simulink model "Alex_SERGIO_wrist"  (R2016b)
settings: Solver=FixedStepDiscrete  StartTime=0.0  StopTime=3600  FixedStep=1/1000  RelTol=1e-3  EnableMultiTasking=on
values from neighbouring files (symbols this model uses):
  abs2deg_s1 = (s1max-s1min)/(s1maxabs-s1minabs)    (= 0.280034572169)    [Alex_init_const_wrist.m]
  abs2deg_s2 = (s2max-s2min)/(s2maxabs-s2minabs)    (= 0.060826446281)    [Alex_init_const_wrist.m]
  ilim_w1 = 1.0    (= 1)    [Alex_init_const_wrist.m]
  ilim_w2 = 1.0    (= 1)    [Alex_init_const_wrist.m]
  Kd_w1 = 0.0    (= 0)    [Alex_init_const_wrist.m]
  Kd_w2 = 0.0    (= 0)    [Alex_init_const_wrist.m]
  Ki_w1 = 0.0    (= 0)    [Alex_init_const_wrist.m]
  Ki_w2 = 0.0    (= 0)    [Alex_init_const_wrist.m]
  s1maxabs = 2374    [Alex_init_const_wrist.m]
  s1minabs = 1217    [Alex_init_const_wrist.m]
  s2maxabs = 3420    [Alex_init_const_wrist.m]
  s2minabs = 395    [Alex_init_const_wrist.m]
  Ts = 1/Fs    [Alex_init_const_shoulderelbow.m]    (also in Alex_init_const_wrist.m = 0.001)
undefined symbols (not defined in the file or in its folder): CPT_w1, CPT_w2, GR_w1, GR_w2
libraries: SERGIOarm x4, SERGIO_Lib x1
settings Model: SimulationMode=external  ExtModeTrigElement=1  ExtModeTrigDuration=3910  ExtModeAutoUpdateStatusClock=off  Creator=root  LastModifiedBy=Matthijs
settings DataIOCC: MaxDataPoints=4000*3600  SaveFormat=Array  SignalLoggingSaveFormat=ModelDataLogs  SaveOutput=off  SignalLogging=off  SaveTime=off
settings OptimizationCC: BlockReduction=off  BooleanDataType=off  ExpressionDepthLimit=2147483647  InitFltsAndDblsToZero=on  LifeSpan=inf
settings DebuggingCC: SaveWithParameterizedLinksMsg=none  UnderspecifiedInitializationDetection=Classic  MergeDetectMultiDrivingBlocksExec=none  SignalResolutionControl=TryResolveAllWithWarning  MultiTaskDSMMsg=warning  MultiTaskCondExecSysMsg=none  FcnCallInpInsideContextMsg=warning  StateNameClashWarn=warning  StrictBusMsg=None  SFUnexpectedBacktrackingDiag=warning  SFNoUnconditionalDefaultTransitionDiag=warning  SFExecutionAtInitializationDiag=none
settings HardwareCC: ProdBitPerPointer=32  ProdBitPerSizeT=32  ProdBitPerPtrDiffT=32  ProdLargestAtomicFloat=None  ProdIntDivRoundTo=Undefined  ProdEndianess=Unspecified  ProdWordSize=32  ProdHWDeviceType=32-bit Generic  TargetBitPerPointer=64  TargetBitPerSizeT=64  TargetBitPerPtrDiffT=64  TargetLongLongMode=on  TargetIntDivRoundTo=Zero  TargetEndianess=LittleEndian  TargetWordSize=64  TargetHWDeviceType=MATLAB Host
settings ModelReferenceCC: ModelReferencePassRootInputsByReference=off  PropagateSignalLabelsOutOfModel=off
settings RTWCC: SystemTargetFile=mttarget.tlc  MakeCommand="make_rtw CC=\"ccache gcc\" OPTS=\"-DNETIF_ID=0 -D_GNU_SOURCE -DPRIO=99\""  TemplateMakefile=mt_unix.tmf  Description=Robocup Real-Time Motion Target  RTWCompilerOptimization=Custom  RTWCustomCompilerOptimizations=-O2 -g -W
settings RTWCC: CustomInclude=|
  | /usr/local/include/soem
  | /usr/local/include/timer_posix
settings RTWCC: CustomLibrary=|
  | /usr/local/lib/libsoem.so
  | /usr/lib/libtimer_posix.so
settings GRTTargetCC: TargetLangStandard=C89/C90 (ANSI)  GeneratePreprocessorConditionals=Disable all  UseToolchainInfoCompliant=off  ExtMode=on
settings ConfigComp: CovMetricSettings=dw  CovHtmlReporting=on  CovSaveCumulativeToWorkspaceVar=on  CovSaveSingleToWorkspaceVar=on  CovExternalEMLEnable=off

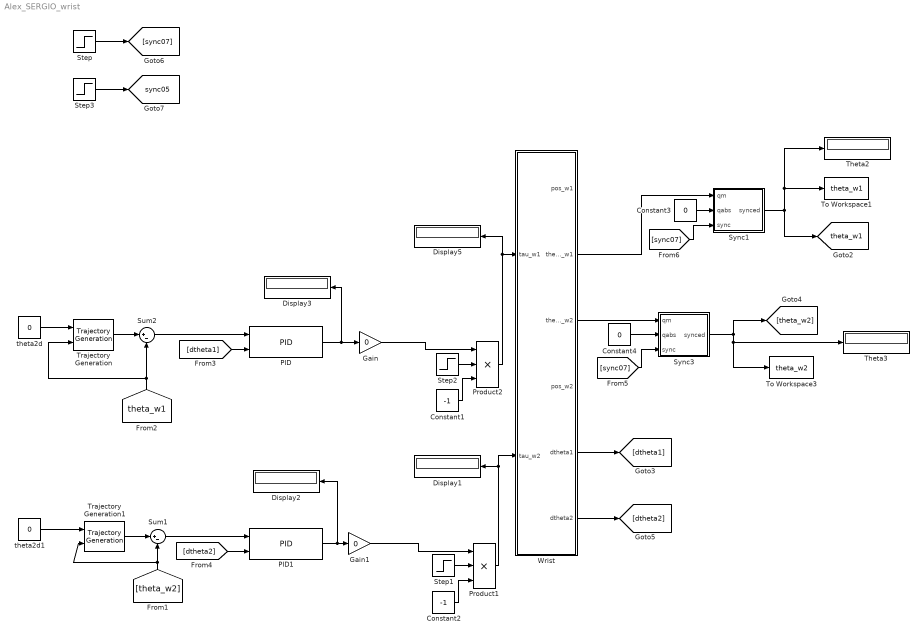
== system Alex_SERGIO_wrist ==
  Constant1 : Constant  Value=-1
  Constant2 : Constant  Value=-1
  Constant3 : Constant  Value=0
  Constant4 : Constant  Value=0
  Display{1..3,5} (4 alike) : Display
  Gain : Gain  Gain=0
  Gain1 : Gain  Gain=0
  PID : SERGIOarm/PID  Kc=Kc_w1  Ki=Ki_w1  Kd=Kd_w1  uplim=ilim_w1  lowlim=-ilim_w1  Ts=Ts
  PID1 : SERGIOarm/PID  Kc=Kc_w2  Ki=Ki_w2  Kd=Kd_w2  uplim=ilim_w2  lowlim=-ilim_w2  Ts=Ts
  Product1 : Product  Inputs=3  RndMeth=Zero
  Product2 : Product  Inputs=3  RndMeth=Zero
  Step : Step  Time=0.7  Before=1  After=0  SampleTime=0
  Step1 : Step  Time=0.8  After=0  SampleTime=0
  Step2 : Step  Time=0.8  After=0  SampleTime=0
  Step3 : Step  Time=0.5  Before=1  After=0  SampleTime=0
  Sum1 : Sum  Inputs=|+-
  Sum2 : Sum  Inputs=|+-
  Sync1 : Subsystem
  Sync3 : Subsystem
  Theta2 : Display
  Theta3 : Display
  To Workspace1 : ToWorkspace  VariableName=theta_w1  SampleTime=-1
  To Workspace3 : ToWorkspace  VariableName=theta_w2  SampleTime=-1
  Trajectory Generation : SERGIOarm/Trajectory Generation  Vmax=0  Amax=0  dif_in=0
  Trajectory Generation1 : SERGIOarm/Trajectory Generation  Vmax=0  Amax=0  dif_in=0
  Wrist : Subsystem
  theta2d : Constant  Value=0
  theta2d1 : Constant  Value=0
  tag scope: sync05=global, theta_w1=global
  wires:
  [theta_w1] -> Sum2/2, Trajectory Generation/2
  Product2/1 -> Wrist/1(tau_w1), Display5/1
  Step/1 -> [sync07]
  Step3/1 -> [sync05]
  Step2/1 -> Product2/2
  Constant1/1 -> Product2/3
  [dtheta1] -> PID/2
  [theta_w2] -> Sum1/2, Trajectory Generation1/2
  Product1/1 -> Display1/1, Wrist/2(tau_w2)
  Step1/1 -> Product1/2
  Constant2/1 -> Product1/3
  [dtheta2] -> PID1/2
  Sync3/1(synced) -> [theta_w2], Theta3/1, To Workspace3/1
  [sync07] -> Sync3/3(sync)
  Sum1/1 -> PID1/1
  [sync07] -> Sync1/3(sync)
  Sync1/1(synced) -> [theta_w1], To Workspace1/1, Theta2/1
  Wrist/2(theta_w1) -> Sync1/1(qm)
  Constant3/1 -> Sync1/2(qabs)
  Wrist/3(theta_w2) -> Sync3/1(qm)
  Constant4/1 -> Sync3/2(qabs)
  Wrist/6(dtheta2) -> [dtheta2]
  Wrist/5(dtheta1) -> [dtheta1]
  PID/1 -> Gain/1, Display3/1
  Gain/1 -> Product2/1
  PID1/1 -> Gain1/1, Display2/1
  Gain1/1 -> Product1/1
  theta2d/1 -> Trajectory Generation/1
  Trajectory Generation/1 -> Sum2/1
  Sum2/1 -> PID/1
  Trajectory Generation1/1 -> Sum1/1
  theta2d1/1 -> Trajectory Generation1/1

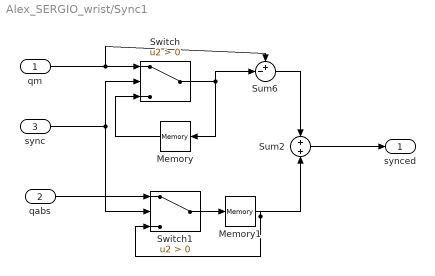
== system Alex_SERGIO_wrist/Sync1 ==
  qm : Inport
  qabs : Inport  Port=2
  sync : Inport  Port=3
  Memory : Memory
  Memory1 : Memory
  Sum2 : Sum
  Sum6 : Sum  Inputs=+-|
  Switch : Switch  Criteria=u2 > Threshold
  Switch1 : Switch  Criteria=u2 > Threshold
  synced : Outport
  wires:
  Switch/1 -> Sum6/2, Memory/1
  Memory/1 -> Switch/3
  qm/1 -> Switch/1, Sum6/1
  Sum6/1 -> Sum2/1
  Sum2/1 -> synced/1
  sync/1 -> Switch/2, Switch1/2
  Memory1/1 -> Switch1/3, Sum2/2
  Switch1/1 -> Memory1/1
  qabs/1 -> Switch1/1

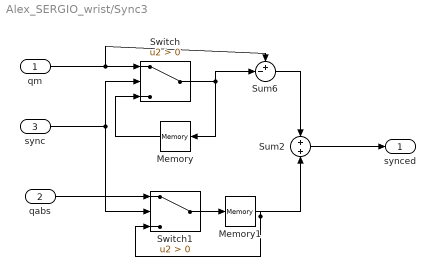
== system Alex_SERGIO_wrist/Sync3 ==
  qm : Inport
  qabs : Inport  Port=2
  sync : Inport  Port=3
  Memory : Memory
  Memory1 : Memory
  Sum2 : Sum
  Sum6 : Sum  Inputs=+-|
  Switch : Switch  Criteria=u2 > Threshold
  Switch1 : Switch  Criteria=u2 > Threshold
  synced : Outport
  wires:
  Switch/1 -> Sum6/2, Memory/1
  Memory/1 -> Switch/3
  qm/1 -> Switch/1, Sum6/1
  Sum6/1 -> Sum2/1
  Sum2/1 -> synced/1
  sync/1 -> Switch/2, Switch1/2
  Memory1/1 -> Switch1/3, Sum2/2
  Switch1/1 -> Memory1/1
  qabs/1 -> Switch1/1

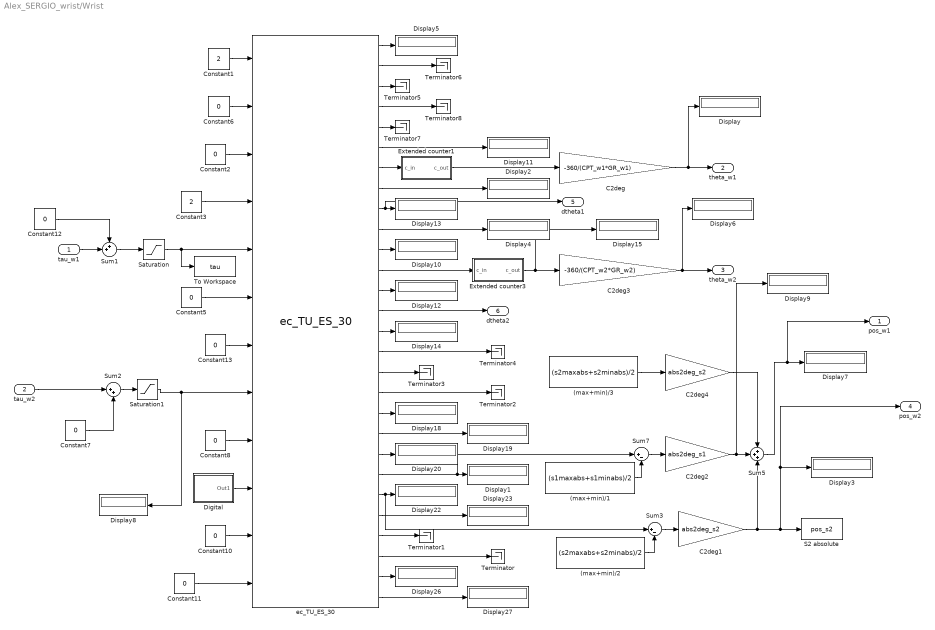
== system Alex_SERGIO_wrist/Wrist ==
  tau_w1 : Inport
  tau_w2 : Inport  Port=2
  (max+min)/1 : Constant  Value=(s1maxabs+s1minabs)/2
  (max+min)/2 : Constant  Value=(s2maxabs+s2minabs)/2
  (max+min)/3 : Constant  Value=(s2maxabs+s2minabs)/2
  C2deg : Gain  Gain=-360/(CPT_w1*GR_w1)
  C2deg1 : Gain  Gain=abs2deg_s2
  C2deg2 : Gain  Gain=abs2deg_s1
  C2deg3 : Gain  Gain=-360/(CPT_w2*GR_w2)
  C2deg4 : Gain  Gain=abs2deg_s2
  Constant1 : Constant  Value=2
  Constant{2,5..8,10..13} (9 alike) : Constant  Value=0
  Constant3 : Constant  Value=2
  Digital : Subsystem
  Display{,1..15,18..20,22..23,26..27} (23 alike) : Display
  Extended counter1 : Subsystem
  Extended counter3 : Subsystem
  S2 absolute : ToWorkspace  VariableName=pos_s2  SampleTime=-1
  Saturation : Saturate  UpperLimit=400  LowerLimit=-400
  Saturation1 : Saturate  UpperLimit=400  LowerLimit=-400
  Sum1 : Sum  Inputs=++|
  Sum2 : Sum  Inputs=|++
  Sum3 : Sum  Inputs=|+-
  Sum5 : Sum  Inputs=+++
  Sum7 : Sum  Inputs=|+-
  Terminator{,1..8} (9 alike) : Terminator
  To Workspace : ToWorkspace  VariableName=tau  SampleTime=-1
  ec_TU_ES_30 : SERGIO_Lib/EtherCAT Blocks/ec_TU_ES_30  link_id=3  slave_num=4  resistance=[0.0, 0, 0]  kv=[0.0, 0, 0]  pgain=[0.00, 10.00, 0.00]  igain=[0.00, 5.00, 0.00]  ilimit=[1.0, 1.0, 1.0]  encdir=[1, 1, -1]  encres=[1024, 512, 512]  czero=[17230, 8835, 8775]
  pos_w1 : Outport
  theta_w1 : Outport  Port=2
  theta_w2 : Outport  Port=3
  pos_w2 : Outport  Port=4
  dtheta1 : Outport  Port=5
  dtheta2 : Outport  Port=6
  wires:
  Constant2/1 -> ec_TU_ES_30/3
  Constant5/1 -> ec_TU_ES_30/6
  Constant8/1 -> ec_TU_ES_30/9
  Digital/1(Out1) -> ec_TU_ES_30/10
  Constant10/1 -> ec_TU_ES_30/11
  Constant11/1 -> ec_TU_ES_30/12
  ec_TU_ES_30/1 -> Display5/1
  ec_TU_ES_30/3 -> Terminator5/1
  ec_TU_ES_30/5 -> Terminator7/1
  ec_TU_ES_30/6 -> Display11/1
  ec_TU_ES_30/8 -> Display2/1
  ec_TU_ES_30/9 -> Display13/1, dtheta1/1
  ec_TU_ES_30/10 -> Display4/1
  ec_TU_ES_30/11 -> Display10/1
  ec_TU_ES_30/13 -> Display12/1
  ec_TU_ES_30/14 -> dtheta2/1
  ec_TU_ES_30/15 -> Display14/1
  ec_TU_ES_30/16 -> Terminator4/1
  ec_TU_ES_30/17 -> Terminator3/1
  ec_TU_ES_30/18 -> Terminator2/1
  ec_TU_ES_30/19 -> Display18/1
  ec_TU_ES_30/20 -> Display19/1
  ec_TU_ES_30/21 -> Display20/1
  ec_TU_ES_30/24 -> Display23/1
  ec_TU_ES_30/25 -> Terminator1/1
  ec_TU_ES_30/26 -> Terminator/1
  ec_TU_ES_30/27 -> Display26/1
  ec_TU_ES_30/28 -> Display27/1
  Sum1/1 -> Saturation/1
  Sum2/1 -> Saturation1/1
  Saturation1/1 -> ec_TU_ES_30/8, Display8/1
  ec_TU_ES_30/7 -> Extended counter1/1(c_in)
  ec_TU_ES_30/12 -> Extended counter3/1(c_in)
  Extended counter3/1(c_out) -> C2deg3/1, Display15/1
  C2deg3/1 -> theta_w2/1, Display6/1
  ec_TU_ES_30/22 -> Display1/1, Sum7/1
  Constant3/1 -> ec_TU_ES_30/4
  Constant12/1 -> Sum1/1
  Constant7/1 -> Sum2/2
  (max+min)/2/1 -> Sum3/2
  Sum3/1 -> C2deg1/1
  C2deg1/1 -> S2 absolute/1, Display3/1, pos_w2/1, Sum5/3
  ec_TU_ES_30/23 -> Display22/1, Sum3/1
  Sum5/1 -> Display7/1, pos_w1/1
  C2deg2/1 -> Display9/1, Sum5/2
  (max+min)/1/1 -> Sum7/2
  Sum7/1 -> C2deg2/1
  (max+min)/3/1 -> C2deg4/1
  C2deg4/1 -> Sum5/1
  Constant1/1 -> ec_TU_ES_30/1
  Constant13/1 -> ec_TU_ES_30/7
  ec_TU_ES_30/2 -> Terminator6/1
  ec_TU_ES_30/4 -> Terminator8/1
  Extended counter1/1(c_out) -> C2deg/1
  C2deg/1 -> theta_w1/1, Display/1
  Saturation/1 -> ec_TU_ES_30/5, To Workspace/1
  Constant6/1 -> ec_TU_ES_30/2
  tau_w1/1 -> Sum1/2
  tau_w2/1 -> Sum2/1

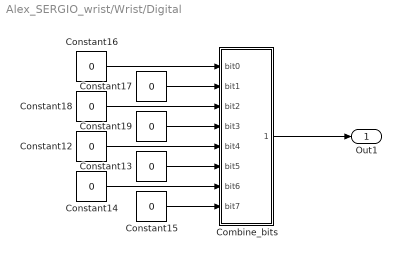
== system Alex_SERGIO_wrist/Wrist/Digital ==
  Combine_bits : Subsystem
  Constant{12..19} (8 alike) : Constant  Value=0
  Out1 : Outport
  wires:
  Constant16/1 -> Combine_bits/1(bit0)
  Constant17/1 -> Combine_bits/2(bit1)
  Constant18/1 -> Combine_bits/3(bit2)
  Constant19/1 -> Combine_bits/4(bit3)
  Constant12/1 -> Combine_bits/5(bit4)
  Constant13/1 -> Combine_bits/6(bit5)
  Constant14/1 -> Combine_bits/7(bit6)
  Constant15/1 -> Combine_bits/8(bit7)
  Combine_bits/1(Out1) -> Out1/1

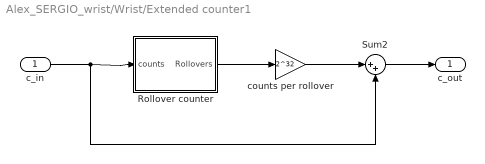
== system Alex_SERGIO_wrist/Wrist/Extended counter1 ==
  c_in : Inport
  Rollover counter : Subsystem
  Sum2 : Sum  Inputs=|++
  counts per rollover : Gain  Gain=2^32
  c_out : Outport
  wires:
  counts per rollover/1 -> Sum2/1
  Rollover counter/1(Rollovers) -> counts per rollover/1
  c_in/1 -> Rollover counter/1(counts), Sum2/2
  Sum2/1 -> c_out/1

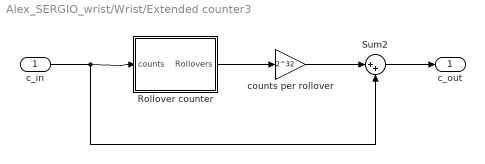
== system Alex_SERGIO_wrist/Wrist/Extended counter3 ==
  c_in : Inport
  Rollover counter : Subsystem
  Sum2 : Sum  Inputs=|++
  counts per rollover : Gain  Gain=2^32
  c_out : Outport
  wires:
  counts per rollover/1 -> Sum2/1
  Rollover counter/1(Rollovers) -> counts per rollover/1
  c_in/1 -> Rollover counter/1(counts), Sum2/2
  Sum2/1 -> c_out/1

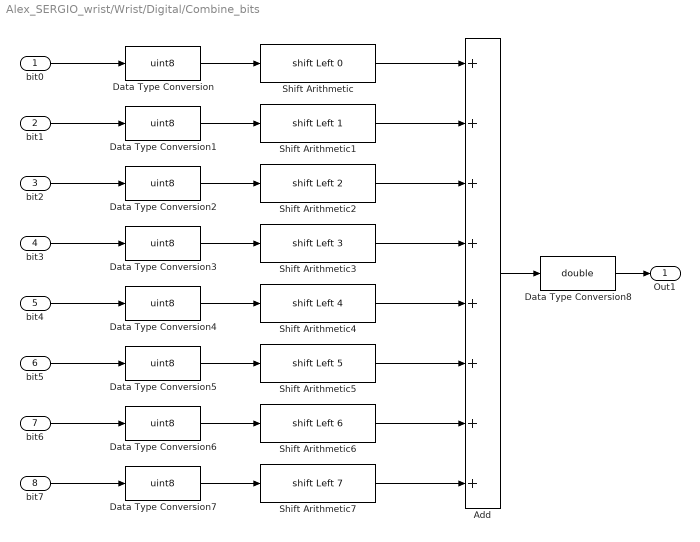
== system Alex_SERGIO_wrist/Wrist/Digital/Combine_bits ==
  bit0 : Inport
  bit1 : Inport  Port=2
  bit2 : Inport  Port=3
  bit3 : Inport  Port=4
  bit4 : Inport  Port=5
  bit5 : Inport  Port=6
  bit6 : Inport  Port=7
  bit7 : Inport  Port=8
  Add : Sum  Inputs=++++++++
  Data Type Conversion{,1..7} (8 alike) : DataTypeConversion  OutDataTypeStr=uint8
  Data Type Conversion8 : DataTypeConversion  OutDataTypeStr=double
  Shift Arithmetic : ArithShift  BitShiftDirection=Left
  Shift Arithmetic1 : ArithShift  BitShiftNumber=1  BitShiftDirection=Left
  Shift Arithmetic2 : ArithShift  BitShiftNumber=2  BitShiftDirection=Left
  Shift Arithmetic3 : ArithShift  BitShiftNumber=3  BitShiftDirection=Left
  Shift Arithmetic4 : ArithShift  BitShiftNumber=4  BitShiftDirection=Left
  Shift Arithmetic5 : ArithShift  BitShiftNumber=5  BitShiftDirection=Left
  Shift Arithmetic6 : ArithShift  BitShiftNumber=6  BitShiftDirection=Left
  Shift Arithmetic7 : ArithShift  BitShiftNumber=7  BitShiftDirection=Left
  Out1 : Outport
  wires:
  bit0/1 -> Data Type Conversion/1
  bit1/1 -> Data Type Conversion1/1
  bit2/1 -> Data Type Conversion2/1
  bit3/1 -> Data Type Conversion3/1
  bit4/1 -> Data Type Conversion4/1
  bit5/1 -> Data Type Conversion5/1
  bit6/1 -> Data Type Conversion6/1
  bit7/1 -> Data Type Conversion7/1
  Data Type Conversion/1 -> Shift Arithmetic/1
  Data Type Conversion1/1 -> Shift Arithmetic1/1
  Data Type Conversion2/1 -> Shift Arithmetic2/1
  Data Type Conversion3/1 -> Shift Arithmetic3/1
  Data Type Conversion4/1 -> Shift Arithmetic4/1
  Data Type Conversion5/1 -> Shift Arithmetic5/1
  Data Type Conversion6/1 -> Shift Arithmetic6/1
  Data Type Conversion7/1 -> Shift Arithmetic7/1
  Shift Arithmetic/1 -> Add/1
  Shift Arithmetic1/1 -> Add/2
  Shift Arithmetic2/1 -> Add/3
  Shift Arithmetic3/1 -> Add/4
  Shift Arithmetic4/1 -> Add/5
  Shift Arithmetic5/1 -> Add/6
  Shift Arithmetic6/1 -> Add/7
  Shift Arithmetic7/1 -> Add/8
  Add/1 -> Data Type Conversion8/1
  Data Type Conversion8/1 -> Out1/1

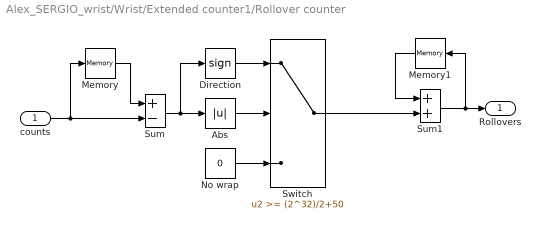
== system Alex_SERGIO_wrist/Wrist/Extended counter1/Rollover counter ==
  counts : Inport
  Abs : Abs
  Direction : Signum
  Memory : Memory  X0=2^32/2  InheritSampleTime=on
  Memory1 : Memory
  No wrap : Constant  Value=0
  Sum : Sum  Inputs=+-
  Sum1 : Sum
  Switch : Switch  Threshold=(2^32)/2+50
  Rollovers : Outport
  wires:
  Memory1/1 -> Sum1/1
  Sum1/1 -> Memory1/1, Rollovers/1
  Switch/1 -> Sum1/2
  Direction/1 -> Switch/1
  No wrap/1 -> Switch/3
  Abs/1 -> Switch/2
  Sum/1 -> Abs/1, Direction/1
  Memory/1 -> Sum/1
  counts/1 -> Sum/2, Memory/1

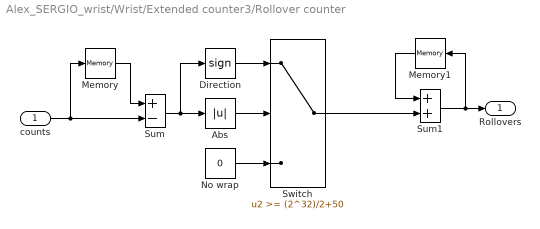
== system Alex_SERGIO_wrist/Wrist/Extended counter3/Rollover counter ==
  counts : Inport
  Abs : Abs
  Direction : Signum
  Memory : Memory  X0=2^32/2  InheritSampleTime=on
  Memory1 : Memory
  No wrap : Constant  Value=0
  Sum : Sum  Inputs=+-
  Sum1 : Sum
  Switch : Switch  Threshold=(2^32)/2+50
  Rollovers : Outport
  wires:
  Memory1/1 -> Sum1/1
  Sum1/1 -> Memory1/1, Rollovers/1
  Switch/1 -> Sum1/2
  Direction/1 -> Switch/1
  No wrap/1 -> Switch/3
  Abs/1 -> Switch/2
  Sum/1 -> Abs/1, Direction/1
  Memory/1 -> Sum/1
  counts/1 -> Sum/2, Memory/1
